simulink model "Ieee14_CC_2019b"  (R2019b)
settings: Solver=ode1  StartTime=0.0  StopTime=3600  FixedStep=1e-3  MaxStep=1e-4  RelTol=1e-3
model workspace (MAT data in the model file):
  pruebaValor = 0
libraries: powerlib x118, dspnetwork x116, source_mod x14, simulink x1
(part 1 of 3)
settings Model: NumberOfSteps=10  OrderedModelArguments=off  Creator=Mónica Alonso  LastModifiedBy=COSEC
settings DataIOCC: ReturnWorkspaceOutputs=off
settings OptimizationCC: LocalBlockOutputs=off
settings DebuggingCC: UnconnectedInputMsg=none  UnconnectedOutputMsg=none  UnconnectedLineMsg=none  ArithmeticOperatorsInVariantConditions=warning
settings SFSimCC: SimUseLocalCustomCode=off  CustomCodeUndefinedFunction=UseInterfaceOnly
settings RTWCC: RTWUseLocalCustomCode=off

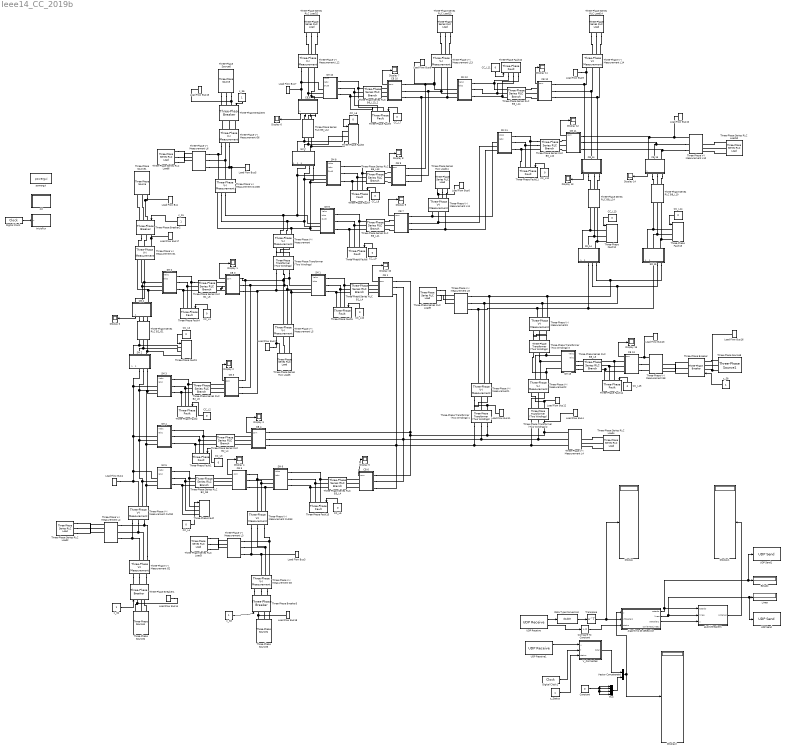
== system Ieee14_CC_2019b ==
  " ajustVBreakers" : MATLAB Function  TreatAsAtomicUnit=on
  "Algoritmo de deteccion " : MATLAB Function  TreatAsAtomicUnit=on
  CB 0 : Subsystem
  CB 1 : Subsystem
  CB 10 : Subsystem
  CB 11 : Subsystem
  CB 12 : Subsystem
  CB 13 : Subsystem
  CB 14 : Subsystem
  CB 15 : Subsystem
  CB 2 : Subsystem
  CB 3 : Subsystem
  CB 4 : Subsystem
  CB 5 : Subsystem
  CB 6 : Subsystem
  CB 7 : Subsystem
  CB 8 : Subsystem
  CB 9 : Subsystem
  CC : MATLAB Function  TreatAsAtomicUnit=on
  CC_L{0..15} (16 alike) : Constant  Value=0
  Compare To Constant : simulink/Logic and Bit Operations/Compare To Constant  relop=>  const=0  OutDataTypeStr=boolean
  Constant : Constant  Value=0
  Data Type Conversion : DataTypeConversion  OutDataTypeStr=double
  Digital Clock : DigitalClock  SampleTime=1e-1
  Digital Clock1 : DigitalClock  SampleTime=1e-3
  Display : Display
  Display {0..15} (16 alike) : Display
      settings: Format=decimal (Stored Integer)
  Display1 : Display
  Display2 : Display
  Estado : Display
  InicioFcn : MATLAB Function  TreatAsAtomicUnit=on
  Linea : Display
  Load Flow Bus : powerlib/Measurements/Load Flow Bus  LConnTagsString=a  Phases=single  Connectors=on one side  ID=BUS_G1  Vbase=69e3  Vref=1.06  Vangle=0  VLF=1.06  VLFb=1  VLFc=1  angleLF=0  angleLFb=0  angleLFc=0
      settings: SourceProductName=Simscape Electrical
  Load Flow Bus1 : powerlib/Measurements/Load Flow Bus  LConnTagsString=a  Phases=single  Connectors=on one side  ID=BUS_2  Vbase=69e3  Vref=1.045  Vangle=0  VLF=1.045  VLFb=1  VLFc=1  angleLF=-0.4295  angleLFb=0  angleLFc=0
      settings: SourceProductName=Simscape Electrical
  Load Flow Bus10 : powerlib/Measurements/Load Flow Bus  LConnTagsString=a  Phases=single  Connectors=on one side  ID=BUS_10  Vbase=13.8e3  Vref=1  Vangle=0  VLF=1.028  VLFb=1  VLFc=1  angleLF=-4.763  angleLFb=0  angleLFc=0
      settings: SourceProductName=Simscape Electrical
  Load Flow Bus11 : powerlib/Measurements/Load Flow Bus  LConnTagsString=a  Phases=single  Connectors=on one side  ID=BUS_9  Vbase=13.8e3  Vref=1  Vangle=0  VLF=1.042  VLFb=1  VLFc=1  angleLF=-4.02  angleLFb=0  angleLFc=0
      settings: SourceProductName=Simscape Electrical
  Load Flow Bus12 : powerlib/Measurements/Load Flow Bus  LConnTagsString=a  Phases=single  Connectors=on one side  ID=BUS_7  Vbase=18e3  Vref=1  Vangle=0  VLF=1.042  VLFb=1  VLFc=1  angleLF=-3.998  angleLFb=0  angleLFc=0
      settings: SourceProductName=Simscape Electrical
  Load Flow Bus13 : powerlib/Measurements/Load Flow Bus  LConnTagsString=a  Phases=single  Connectors=on one side  ID=BUS_8  Vbase=18e3  Vref=1.09  Vangle=0  VLF=1.082  VLFb=1  VLFc=1  angleLF=-4.037  angleLFb=0  angleLFc=0
      settings: SourceProductName=Simscape Electrical
  Load Flow Bus14 : powerlib/Measurements/Load Flow Bus  LConnTagsString=a  Phases=single  Connectors=on one side  ID=BUS_G2  Vbase=69e3  Vref=1.045  Vangle=0  VLF=1.045  VLFb=1  VLFc=1  angleLF=-0.435  angleLFb=0  angleLFc=0
      settings: SourceProductName=Simscape Electrical
  Load Flow Bus15 : powerlib/Measurements/Load Flow Bus  LConnTagsString=a  Phases=single  Connectors=on one side  ID=BUS_G6  Vbase=13.8e3  Vref=1.07  Vangle=0  VLF=1.07  VLFb=1  VLFc=1  angleLF=-4.448  angleLFb=0  angleLFc=0
      settings: SourceProductName=Simscape Electrical
  Load Flow Bus16 : powerlib/Measurements/Load Flow Bus  LConnTagsString=a  Phases=single  Connectors=on one side  ID=BUS_G8  Vbase=18e3  Vref=1.09  Vangle=0  VLF=1.082  VLFb=1  VLFc=1  angleLF=-4.074  angleLFb=0  angleLFc=0
      settings: SourceProductName=Simscape Electrical
  Load Flow Bus17 : powerlib/Measurements/Load Flow Bus  LConnTagsString=a  Phases=single  Connectors=on one side  ID=BUS_1  Vbase=69e3  Vref=1.06  Vangle=0  VLF=1.06  VLFb=1  VLFc=1  angleLF=0.000603  angleLFb=0  angleLFc=0
      settings: SourceProductName=Simscape Electrical
  Load Flow Bus18 : powerlib/Measurements/Load Flow Bus  LConnTagsString=a  Phases=single  Connectors=on one side  ID=BUS_G3  Vbase=69e3  Vref=1.01  Vangle=0  VLF=1.029  VLFb=1  VLFc=1  angleLF=-1.19  angleLFb=0  angleLFc=0
      settings: SourceProductName=Simscape Electrical
  Load Flow Bus2 : powerlib/Measurements/Load Flow Bus  LConnTagsString=a  Phases=single  Connectors=on one side  ID=BUS_5  Vbase=69e3  Vref=1  Vangle=0  VLF=1.008  VLFb=1  VLFc=1  angleLF=-3.193  angleLFb=0  angleLFc=0
      settings: SourceProductName=Simscape Electrical
  Load Flow Bus3 : powerlib/Measurements/Load Flow Bus  LConnTagsString=a  Phases=single  Connectors=on one side  ID=BUS_3  Vbase=69e3  Vref=1.01  Vangle=0  VLF=1.029  VLFb=1  VLFc=1  angleLF=-1.19  angleLFb=0  angleLFc=0
      settings: SourceProductName=Simscape Electrical
  Load Flow Bus4 : powerlib/Measurements/Load Flow Bus  LConnTagsString=a  Phases=single  Connectors=on one side  ID=BUS_4  Vbase=69e3  Vref=1  Vangle=0  VLF=1.013  VLFb=1  VLFc=1  angleLF=-3.392  angleLFb=0  angleLFc=0
      settings: SourceProductName=Simscape Electrical
  Load Flow Bus5 : powerlib/Measurements/Load Flow Bus  LConnTagsString=a  Phases=single  Connectors=on one side  ID=BUS_6  Vbase=13.8e3  Vref=1.07  Vangle=0  VLF=1.07  VLFb=1  VLFc=1  angleLF=-4.411  angleLFb=0  angleLFc=0
      settings: SourceProductName=Simscape Electrical
  Load Flow Bus6 : powerlib/Measurements/Load Flow Bus  LConnTagsString=a  Phases=single  Connectors=on one side  ID=BUS_11  Vbase=13.8e3  Vref=1  Vangle=0  VLF=1.029  VLFb=1  VLFc=1  angleLF=-5.425  angleLFb=0  angleLFc=0
      settings: SourceProductName=Simscape Electrical
  Load Flow Bus7 : powerlib/Measurements/Load Flow Bus  LConnTagsString=a  Phases=single  Connectors=on one side  ID=BUS_12  Vbase=13.8e3  Vref=1  Vangle=0  VLF=1.034  VLFb=1  VLFc=1  angleLF=-5.514  angleLFb=0  angleLFc=0
      settings: SourceProductName=Simscape Electrical
  Load Flow Bus8 : powerlib/Measurements/Load Flow Bus  LConnTagsString=a  Phases=single  Connectors=on one side  ID=BUS_13  Vbase=13.8e3  Vref=1  Vangle=0  VLF=1.036  VLFb=1  VLFc=1  angleLF=-5.353  angleLFb=0  angleLFc=0
      settings: SourceProductName=Simscape Electrical
  Load Flow Bus9 : powerlib/Measurements/Load Flow Bus  LConnTagsString=a  Phases=single  Connectors=on one side  ID=BUS_14  Vbase=13.8e3  Vref=1  Vangle=0  VLF=1.013  VLFb=1  VLFc=1  angleLF=-5.548  angleLFb=0  angleLFc=0
      settings: SourceProductName=Simscape Electrical
  Mux : Mux
  SM 0 : Subsystem
  SM 1 : Subsystem
  SM 10 : Subsystem
  SM 11 : Subsystem
  SM 12 : Subsystem
  SM 13 : Subsystem
  SM 14 : Subsystem
  SM 15 : Subsystem
  SM 2 : Subsystem
  SM 3 : Subsystem
  SM 4 : Subsystem
  SM 5 : Subsystem
  SM 6 : Subsystem
  SM 7 : Subsystem
  SM 8 : Subsystem
  SM 9 : Subsystem
  Three-Phase Series RLC B1_L4 : powerlib/Elements/Three-Phase Series RLC Branch  LConnTagsString=A|B|C  RConnTagsString=A|B|C  BranchType=RL  Resistance=0.01335*47.61  Inductance=0.04211*47.61/(100*pi)  Capacitance=100*pi/0.034  Measurements=None
      settings: SourceProductName=Simscape Electrical
  Three-Phase Series RLC B1_L5 : powerlib/Elements/Three-Phase Series RLC Branch  LConnTagsString=A|B|C  RConnTagsString=A|B|C  BranchType=RLC  Resistance=0.05403*47.61  Inductance=0.22304*47.61/(100*pi)  Capacitance=1/(0.0492*47.61*100*pi)  Measurements=None
      settings: SourceProductName=Simscape Electrical
  Three-Phase Series RLC B2_G1 : powerlib/Elements/Three-Phase Series RLC Branch  LConnTagsString=A|B|C  RConnTagsString=A|B|C  BranchType=RLC  Resistance=0.01938*47.61  Inductance=0.05917*47.61/(100*pi)  Capacitance=1/(0.0528*47.61*100*pi)  Measurements=None
      settings: SourceProductName=Simscape Electrical
  Three-Phase Series RLC B2_G3 : powerlib/Elements/Three-Phase Series RLC Branch  LConnTagsString=A|B|C  RConnTagsString=A|B|C  BranchType=RLC  Resistance=0.04699*47.61  Inductance=0.19797*47.61/(100*pi)  Capacitance=1/(0.0438*47.61*100*pi)  Measurements=None
      settings: SourceProductName=Simscape Electrical
  Three-Phase Series RLC B2_L4 : powerlib/Elements/Three-Phase Series RLC Branch  LConnTagsString=A|B|C  RConnTagsString=A|B|C  BranchType=RLC  Resistance=0.05811*47.61  Inductance=0.17632*47.61/(100*pi)  Capacitance=1/(0.034*47.61*100*pi)  Measurements=None
      settings: SourceProductName=Simscape Electrical
  Three-Phase Series RLC B2_L5 : powerlib/Elements/Three-Phase Series RLC Branch  LConnTagsString=A|B|C  RConnTagsString=A|B|C  BranchType=RLC  Resistance=0.05695*47.61  Inductance=0.17388*47.61/(100*pi)  Capacitance=1/(0.0346*47.61*100*pi)  Measurements=None
      settings: SourceProductName=Simscape Electrical
  Three-Phase Series RLC B3_L4 : powerlib/Elements/Three-Phase Series RLC Branch  LConnTagsString=A|B|C  RConnTagsString=A|B|C  BranchType=RLC  Resistance=0.06701*47.61  Inductance=0.17103*47.61/(100*pi)  Capacitance=1/(0.0128*47.61*100*pi)  Measurements=None
      settings: SourceProductName=Simscape Electrical
  Three-Phase Series RLC B6_L10 : powerlib/Elements/Three-Phase Series RLC Branch  LConnTagsString=A|B|C  RConnTagsString=A|B|C  BranchType=RL  Resistance=0.17093*1.9044  Inductance=0.34802*1.9044/(100*pi)  Capacitance=100*pi/0.034  Measurements=None
      settings: SourceProductName=Simscape Electrical
  Three-Phase Series RLC B6_L11 : powerlib/Elements/Three-Phase Series RLC Branch  LConnTagsString=A|B|C  RConnTagsString=A|B|C  BranchType=RL  Resistance=0.09498*1.9044  Inductance=0.1989*1.9044/(100*pi)  Capacitance=100*pi/0.034  Measurements=None
      settings: SourceProductName=Simscape Electrical
  Three-Phase Series RLC B6_L12 : powerlib/Elements/Three-Phase Series RLC Branch  LConnTagsString=A|B|C  RConnTagsString=A|B|C  BranchType=RL  Resistance=0.12291*1.9044  Inductance=0.25581*1.9044/(100*pi)  Capacitance=100*pi/0.034  Measurements=None
      settings: SourceProductName=Simscape Electrical
  Three-Phase Series RLC B6_L13 : powerlib/Elements/Three-Phase Series RLC Branch  LConnTagsString=A|B|C  RConnTagsString=A|B|C  BranchType=RL  Resistance=0.06615*1.9044  Inductance=0.13027*1.9044/(100*pi)  Capacitance=100*pi/0.034  Measurements=None
      settings: SourceProductName=Simscape Electrical
  Three-Phase Series RLC B6_L13_2 : powerlib/Elements/Three-Phase Series RLC Branch  LConnTagsString=A|B|C  RConnTagsString=A|B|C  BranchType=RL  Resistance=0.06615*1.9044  Inductance=0.13027*1.9044/(100*pi)  Capacitance=100*pi/0.034  Measurements=None
      settings: SourceProductName=Simscape Electrical
  Three-Phase Series RLC B6_L14 : powerlib/Elements/Three-Phase Series RLC Branch  LConnTagsString=A|B|C  RConnTagsString=A|B|C  BranchType=RL  Resistance=0.17093*1.9044  Inductance=0.34802*1.9044/(100*pi)  Capacitance=100*pi/0.034  Measurements=None
      settings: SourceProductName=Simscape Electrical
  Three-Phase Series RLC B8_L10 : powerlib/Elements/Three-Phase Series RLC Branch  LConnTagsString=A|B|C  RConnTagsString=A|B|C  BranchType=RL  Resistance=0.03181*1.9044  Inductance=0.0845*1.9044/(100*pi)  Capacitance=100*pi/0.034  Measurements=None
      settings: SourceProductName=Simscape Electrical
  Three-Phase Series RLC B8_L14 : powerlib/Elements/Three-Phase Series RLC Branch  LConnTagsString=A|B|C  RConnTagsString=A|B|C  BranchType=RL  Resistance=0.12711*1.9044  Inductance=0.27038*1.9044/(100*pi)  Capacitance=100*pi/0.034  Measurements=None
      settings: SourceProductName=Simscape Electrical
  Three-Phase Series RLC B8_L5 : powerlib/Elements/Three-Phase Series RLC Branch  LConnTagsString=A|B|C  RConnTagsString=A|B|C  BranchType=L  Resistance=0  Inductance=0.17615*3.24/(100*pi)  Capacitance=100*pi/0.034  Measurements=None
      settings: SourceProductName=Simscape Electrical
  Three-Phase Series RLC Load10 : source_mod/Three-Phase Series RLC Load  LConnTagsString=A|B|C  Configuration=Y (grounded)  NominalVoltage=(13800)*1.028  Vabc=[1e3 1e3 1e3]  Vabcp=[1e3 1e3 1e3]  NominalFrequency=50  UnbalancedPower=off  ActivePower=17472840  InductivePower=10226040  CapacitivePower=100  Pabc=[10e3 9e3 11e3]  QLabc=[100 90 110]  QCabc=[100 90 110]  Pabcp=[10e3 9e3 11e3]  QLabcp=[100 90 110]  QCabcp=[100 90 110]  Measurements=Branch voltages and currents  LoadType=constant PQ
      settings: AttributesFormatString=\n  SourceProductName=my library
  Three-Phase Series RLC Load11 : source_mod/Three-Phase Series RLC Load  LConnTagsString=A|B|C  Configuration=Y (grounded)  NominalVoltage=(13800)*1.02933  Vabc=[1e3 1e3 1e3]  Vabcp=[1e3 1e3 1e3]  NominalFrequency=50  UnbalancedPower=off  ActivePower=14912240  InductivePower=8727440  CapacitivePower=0  Pabc=[10e3 9e3 11e3]  QLabc=[100 90 110]  QCabc=[100 90 110]  Pabcp=[10e3 9e3 11e3]  QLabcp=[100 90 110]  QCabcp=[100 90 110]  Measurements=Branch voltages and currents  LoadType=constant PQ
      settings: AttributesFormatString=\n  SourceProductName=my library
  Three-Phase Series RLC Load12 : source_mod/Three-Phase Series RLC Load  LConnTagsString=A|B|C  Configuration=Y (grounded)  NominalVoltage=(13800)*1.03362  Vabc=[1e3 1e3 1e3]  Vabcp=[1e3 1e3 1e3]  NominalFrequency=50  UnbalancedPower=off  ActivePower=14706090  InductivePower=8606790  CapacitivePower=100  Pabc=[10e3 9e3 11e3]  QLabc=[100 90 110]  QCabc=[100 90 110]  Pabcp=[10e3 9e3 11e3]  QLabcp=[100 90 110]  QCabcp=[100 90 110]  Measurements=Branch voltages and currents  LoadType=constant PQ
      settings: AttributesFormatString=\n  SourceProductName=my library
  Three-Phase Series RLC Load13 : source_mod/Three-Phase Series RLC Load  LConnTagsString=A|B|C  Configuration=Y (grounded)  NominalVoltage=(13800)*1.03599  Vabc=[1e3 1e3 1e3]  Vabcp=[1e3 1e3 1e3]  NominalFrequency=50  UnbalancedPower=off  ActivePower=18199790  InductivePower=10651490  CapacitivePower=100  Pabc=[10e3 9e3 11e3]  QLabc=[100 90 110]  QCabc=[100 90 110]  Pabcp=[10e3 9e3 11e3]  QLabcp=[100 90 110]  QCabcp=[100 90 110]  Measurements=Branch voltages and currents  LoadType=constant PQ
      settings: AttributesFormatString=\n  SourceProductName=my library
  Three-Phase Series RLC Load14 : source_mod/Three-Phase Series RLC Load  LConnTagsString=A|B|C  Configuration=Y (grounded)  NominalVoltage=(13800)*1.01323  Vabc=[1e3 1e3 1e3]  Vabcp=[1e3 1e3 1e3]  NominalFrequency=50  UnbalancedPower=off  ActivePower=13888000  InductivePower=8128000  CapacitivePower=1  Pabc=[10e3 9e3 11e3]  QLabc=[100 90 110]  QCabc=[100 90 110]  Pabcp=[10e3 9e3 11e3]  QLabcp=[100 90 110]  QCabcp=[100 90 110]  Measurements=Branch voltages and currents  LoadType=constant PQ
      settings: AttributesFormatString=\n  SourceProductName=my library
  Three-Phase Series RLC Load2 : source_mod/Three-Phase Series RLC Load  LConnTagsString=A|B|C  Configuration=Y (grounded)  NominalVoltage=(69000)*1.04466  Vabc=[1e3 1e3 1e3]  Vabcp=[1e3 1e3 1e3]  NominalFrequency=50  UnbalancedPower=off  ActivePower=11817820  InductivePower=6916420  CapacitivePower=0  Pabc=15  QLabc=[100 90 110]  QCabc=[100 90 110]  Pabcp=[10e3 9e3 11e3]  QLabcp=[100 90 110]  QCabcp=[100 90 110]  Measurements=Branch voltages and currents  LoadType=constant PQ
      settings: AttributesFormatString=\n  SourceProductName=my library
  Three-Phase Series RLC Load3 : source_mod/Three-Phase Series RLC Load  LConnTagsString=A|B|C  Configuration=Y (grounded)  NominalVoltage=(69000)*1.02865  Vabc=[1e3 1e3 1e3]  Vabcp=[1e3 1e3 1e3]  NominalFrequency=50  UnbalancedPower=off  ActivePower=15090180  InductivePower=8831580  CapacitivePower=0  Pabc=[10e3 9e3 11e3]  QLabc=[100 90 110]  QCabc=[100 90 110]  Pabcp=[10e3 9e3 11e3]  QLabcp=[100 90 110]  QCabcp=[100 90 110]  Measurements=Branch voltages and currents  LoadType=constant PQ
      settings: AttributesFormatString=\n  SourceProductName=my library
  Three-Phase Series RLC Load4 : source_mod/Three-Phase Series RLC Load  LConnTagsString=A|B|C  Configuration=Y (grounded)  NominalVoltage=(69000)*1.0131  Vabc=[1e3 1e3 1e3]  Vabcp=[1e3 1e3 1e3]  NominalFrequency=50  UnbalancedPower=off  ActivePower=20484800  InductivePower=11988800  CapacitivePower=3.9e6  Pabc=[10e3 9e3 11e3]  QLabc=[100 90 110]  QCabc=[100 90 110]  Pabcp=[10e3 9e3 11e3]  QLabcp=[100 90 110]  QCabcp=[100 90 110]  Measurements=Branch voltages and currents  LoadType=constant PQ
      settings: AttributesFormatString=\n  SourceProductName=my library
  Three-Phase Series RLC Load5 : source_mod/Three-Phase Series RLC Load  LConnTagsString=A|B|C  Configuration=Y (grounded)  NominalVoltage=(69000)*1.00791  Vabc=[1e3 1e3 1e3]  Vabcp=[1e3 1e3 1e3]  NominalFrequency=50  UnbalancedPower=off  ActivePower=19805590  InductivePower=11591290  CapacitivePower=0  Pabc=[10e3 9e3 11e3]  QLabc=[100 90 110]  QCabc=[100 90 110]  Pabcp=[10e3 9e3 11e3]  QLabcp=[100 90 110]  QCabcp=[100 90 110]  Measurements=Branch voltages and currents  LoadType=constant PQ
      settings: AttributesFormatString=\n  SourceProductName=my library
  Three-Phase Series RLC Load6 : source_mod/Three-Phase Series RLC Load  LConnTagsString=A|B|C  Configuration=Y (grounded)  NominalVoltage=(13800)*1.07  Vabc=[1e3 1e3 1e3]  Vabcp=[1e3 1e3 1e3]  NominalFrequency=50  UnbalancedPower=off  ActivePower=16845710  InductivePower=9859010  CapacitivePower=0  Pabc=[10e3 9e3 11e3]  QLabc=[100 90 110]  QCabc=[100 90 110]  Pabcp=[10e3 9e3 11e3]  QLabcp=[100 90 110]  QCabcp=[100 90 110]  Measurements=Branch voltages and currents  LoadType=constant PQ
      settings: AttributesFormatString=\n  SourceProductName=my library
  Three-Phase Series RLC Load9 : source_mod/Three-Phase Series RLC Load  LConnTagsString=A|B|C  Configuration=Y (grounded)  NominalVoltage=(13800)*1.04242  Vabc=[1e3 1e3 1e3]  Vabcp=[1e3 1e3 1e3]  NominalFrequency=50  UnbalancedPower=off  ActivePower=12028310  InductivePower=7039610  CapacitivePower=19e6  Pabc=[10e3 9e3 11e3]  QLabc=[100 90 110]  QCabc=[100 90 110]  Pabcp=[10e3 9e3 11e3]  QLabcp=[100 90 110]  QCabcp=[100 90 110]  Measurements=Branch voltages and currents  LoadType=constant PQ
      settings: AttributesFormatString=\n  SourceProductName=my library
  Three-Phase Transformer (Two Windings) : powerlib/Elements/Three-Phase Transformer (Two Windings)  Winding1Connection=Yg  Winding2Connection=Yg  CoreType=Three single-phase transformers  SetSaturation=off  Hysteresis=off  DataFile='hysteresis'  SetInitialFlux=off  Measurements=None  UNITS=pu  NominalPower=[ 100e6 , 50 ]  Winding1="[13.8e3 , 0 ,  0]"  Winding2=[69e3*0.932, 0 ,0.25202*47.61/(100*pi) ]  Rm=500  Lm=500  L0=0.5  Saturation=[ 0,0 ; 0.0024,1.2 ; 1.0,1.52 ]  InitialFluxes=[ 0.8 , -0.8 , 0.7 ]  BreakLoop=off  DiscreteSolver=Trapezoidal iterative  DataType=off  TransfoNumber=1
      settings: SourceProductName=Simscape Electrical
  Three-Phase Transformer (Two Windings)1 : powerlib/Elements/Three-Phase Transformer (Two Windings)  Winding1Connection=Yg  Winding2Connection=Yg  CoreType=Three single-phase transformers  SetSaturation=off  Hysteresis=off  DataFile='hysteresis'  SetInitialFlux=off  Measurements=None  UNITS=pu  NominalPower=[ 100e6 , 50 ]  Winding1=[13.8e3 , 0 , 0 ]  Winding2=[69e3*0.969, 0 , 0.55618*47.61/(100*pi)]  Rm=500  Lm=500  L0=0.5  Saturation=[ 0,0 ; 0.0024,1.2 ; 1.0,1.52 ]  InitialFluxes=[ 0.8 , -0.8 , 0.7 ]  BreakLoop=off  DiscreteSolver=Trapezoidal iterative  DataType=off  TransfoNumber=1
      settings: SourceProductName=Simscape Electrical
  Three-Phase Transformer (Two Windings)2 : powerlib/Elements/Three-Phase Transformer (Two Windings)  Winding1Connection=Yg  Winding2Connection=Yg  CoreType=Three single-phase transformers  SetSaturation=off  Hysteresis=off  DataFile='hysteresis'  SetInitialFlux=off  Measurements=None  UNITS=pu  NominalPower=[ 100e6 , 50 ]  Winding1=[18e3 , 0 , 0]  Winding2=[69e3*0.978 , 0 ,0.20912*47.61/(100*pi)]  Rm=500  Lm=500  L0=0.5  Saturation=[ 0,0 ; 0.0024,1.2 ; 1.0,1.52 ]  InitialFluxes=[ 0.8 , -0.8 , 0.7 ]  BreakLoop=off  DiscreteSolver=Trapezoidal iterative  DataType=off  TransfoNumber=1
      settings: SourceProductName=Simscape Electrical
  Three-Phase Transformer (Two Windings)3 : powerlib/Elements/Three-Phase Transformer (Two Windings)  Winding1Connection=Yg  Winding2Connection=Yg  CoreType=Three single-phase transformers  SetSaturation=off  Hysteresis=off  DataFile='hysteresis'  SetInitialFlux=off  Measurements=None  UNITS=pu  NominalPower=[ 100e6 , 50 ]  Winding1=[13.8e3 , 0 , 0]  Winding2=[18e3, 0 ,0.11*3.24/(100*pi)]  Rm=500  Lm=500  L0=0.5  Saturation=[ 0,0 ; 0.0024,1.2 ; 1.0,1.52 ]  InitialFluxes=[ 0.8 , -0.8 , 0.7 ]  BreakLoop=off  DiscreteSolver=Trapezoidal iterative  DataType=off  TransfoNumber=1
      settings: SourceProductName=Simscape Electrical
  Three-Phase V-I Measurement{,1..3} (4 alike) : powerlib/Measurements/Three-Phase V-I Measurement  VoltageMeasurement=no  SetLabelV=off  LabelV=Vabc  Vpu=off  VpuLL=off  CurrentMeasurement=yes  SetLabelI=off  LabelI=Iabc  Ipu=off  Pbase=100e6  Vbase=500e3  OutputType=Complex  PhasorSimulation=off  PSBequivalent=0
      settings: SourceProductName=Simscape Electrical
  Three-Phase V-I Measurement G1 : powerlib/Measurements/Three-Phase V-I Measurement  VoltageMeasurement=phase-to-phase  SetLabelV=off  LabelV=Vabc  Vpu=off  VpuLL=off  CurrentMeasurement=yes  SetLabelI=off  LabelI=Iabc  Ipu=off  Pbase=100e6  Vbase=69e3  OutputType=Complex  PhasorSimulation=off  PSBequivalent=0
      settings: SourceProductName=Simscape Electrical
  Three-Phase V-I Measurement G2 : powerlib/Measurements/Three-Phase V-I Measurement  VoltageMeasurement=phase-to-ground  SetLabelV=off  LabelV=Vabc  Vpu=off  VpuLL=off  CurrentMeasurement=yes  SetLabelI=off  LabelI=Iabc  Ipu=off  Pbase=100e6  Vbase=69e3  OutputType=Complex  PhasorSimulation=off  PSBequivalent=0
      settings: SourceProductName=Simscape Electrical
  Three-Phase V-I Measurement G3 : powerlib/Measurements/Three-Phase V-I Measurement  VoltageMeasurement=phase-to-phase  SetLabelV=off  LabelV=Vabc  Vpu=off  VpuLL=off  CurrentMeasurement=yes  SetLabelI=off  LabelI=Iabc  Ipu=off  Pbase=100e6  Vbase=69e3  OutputType=Complex  PhasorSimulation=off  PSBequivalent=0
      settings: SourceProductName=Simscape Electrical
  Three-Phase V-I Measurement G6 : powerlib/Measurements/Three-Phase V-I Measurement  VoltageMeasurement=phase-to-phase  SetLabelV=off  LabelV=Vabc  Vpu=off  VpuLL=off  CurrentMeasurement=yes  SetLabelI=off  LabelI=Iabc  Ipu=off  Pbase=100e6  Vbase=13.8e3  OutputType=Complex  PhasorSimulation=off  PSBequivalent=0
      settings: SourceProductName=Simscape Electrical
  Three-Phase V-I Measurement G8 : powerlib/Measurements/Three-Phase V-I Measurement  VoltageMeasurement=phase-to-phase  SetLabelV=off  LabelV=Vabc  Vpu=off  VpuLL=off  CurrentMeasurement=yes  SetLabelI=off  LabelI=Iabc  Ipu=off  Pbase=100e6  Vbase=18e3  OutputType=Complex  PhasorSimulation=off  PSBequivalent=0
      settings: SourceProductName=Simscape Electrical
  Three-Phase V-I Measurement L{6,10..14} (6 alike) : powerlib/Measurements/Three-Phase V-I Measurement  VoltageMeasurement=phase-to-phase  SetLabelV=off  LabelV=Vabc  Vpu=off  VpuLL=off  CurrentMeasurement=yes  SetLabelI=off  LabelI=Iabc  Ipu=off  Pbase=100e6  Vbase=13.8e3  OutputType=Complex  PhasorSimulation=off  PSBequivalent=0
      settings: SourceProductName=Simscape Electrical
  Three-Phase V-I Measurement L2 : powerlib/Measurements/Three-Phase V-I Measurement  VoltageMeasurement=phase-to-ground  SetLabelV=off  LabelV=Vabc  Vpu=off  VpuLL=off  CurrentMeasurement=yes  SetLabelI=off  LabelI=Iabc  Ipu=off  Pbase=100e6  Vbase=69e3  OutputType=Complex  PhasorSimulation=off  PSBequivalent=0
      settings: SourceProductName=Simscape Electrical
  Three-Phase V-I Measurement L{3..5,9} (4 alike) : powerlib/Measurements/Three-Phase V-I Measurement  VoltageMeasurement=phase-to-phase  SetLabelV=off  LabelV=Vabc  Vpu=off  VpuLL=off  CurrentMeasurement=yes  SetLabelI=off  LabelI=Iabc  Ipu=off  Pbase=100e6  Vbase=69e3  OutputType=Complex  PhasorSimulation=off  PSBequivalent=0
      settings: SourceProductName=Simscape Electrical
  Three-Phase V-I Measurement OutG2 : powerlib/Measurements/Three-Phase V-I Measurement  VoltageMeasurement=phase-to-phase  SetLabelV=off  LabelV=Vabc  Vpu=on  VpuLL=off  CurrentMeasurement=yes  SetLabelI=off  LabelI=Iabc  Ipu=off  Pbase=100e6  Vbase=69e3  OutputType=Complex  PhasorSimulation=off  PSBequivalent=0
      settings: SourceProductName=Simscape Electrical
  Three-Phase V-I Measurement OutG3 : powerlib/Measurements/Three-Phase V-I Measurement  VoltageMeasurement=phase-to-phase  SetLabelV=off  LabelV=Vabc  Vpu=on  VpuLL=off  CurrentMeasurement=yes  SetLabelI=off  LabelI=Iabc  Ipu=off  Pbase=100e6  Vbase=69e3  OutputType=Complex  PhasorSimulation=off  PSBequivalent=0
      settings: SourceProductName=Simscape Electrical
  Three-Phase V-I Measurement OutG6 : powerlib/Measurements/Three-Phase V-I Measurement  VoltageMeasurement=phase-to-phase  SetLabelV=off  LabelV=Vabc  Vpu=on  VpuLL=off  CurrentMeasurement=yes  SetLabelI=off  LabelI=Iabc  Ipu=off  Pbase=100e6  Vbase=13.8e3  OutputType=Complex  PhasorSimulation=off  PSBequivalent=0
      settings: SourceProductName=Simscape Electrical
  Three-Phase Breaker : powerlib/Elements/Three-Phase Breaker  InitialState=closed  SwitchA=on  SwitchB=on  SwitchC=on  SwitchTimes=[1.5]  External=on  BreakerResistance=0.01  SnubberResistance=1e6  SnubberCapacitance=inf  Measurements=Breaker voltages and currents
      settings: SourceProductName=Simscape Electrical
  Three-Phase Breaker{1..3,6} (4 alike) : powerlib/Elements/Three-Phase Breaker  InitialState=closed  SwitchA=on  SwitchB=on  SwitchC=on  SwitchTimes=[1]  External=on  BreakerResistance=0.01  SnubberResistance=1e6  SnubberCapacitance=inf  Measurements=Breaker voltages and currents
      settings: SourceProductName=Simscape Electrical
  Three-Phase Fault{,1..15} (16 alike) : powerlib/Elements/Three-Phase Fault  InitialStates=0  FaultA=on  FaultB=on  FaultC=on  GroundFault=on  SwitchTimes="[1/60  5/60]"  External=on  SwitchStatus=NaN  FaultResistance=0.001  GroundResistance=0.01  SnubberResistance=1e6  SnubberCapacitance=inf  Measurements=Fault voltages and currents
      settings: SourceProductName=Simscape Electrical
  Three-Phase Source1 : powerlib/Electrical Sources/Three-Phase Source  InternalConnection=Yg  VoltagePhases=off  Voltage=(69000)*1.06  PhaseAngle=0  Voltage_phases=[25e3 25e3 25e3]/sqrt(3)  PhaseAngles_phases=[0 -120 +120]  Frequency=50  NonIdealSource=off  SpecifyImpedance=off  Resistance=0.8929  Inductance=16.58e-3  ShortCircuitLevel=100e6  BaseVoltage=69e3  XRratio=7  BusType=swing  Pref=10e3  Qref=0  Prefabc=[10e3, 10e3, 10e3]  Qrefabc=[0, 0, 0]  Qmin=-inf  Qmax=inf
      settings: SourceProductName=Simscape Electrical
  Three-Phase Source2 : source_mod/Three-Phase Source1  InternalConnection=Yg  VoltagePhases=off  Voltage=(69000)*1.04471  PhaseAngle=-0.43499  Voltage_phases=[25e3 25e3 25e3]/sqrt(3)  PhaseAngles_phases=[0 -120 +120]  Frequency=50  NonIdealSource=off  SpecifyImpedance=on  Resistance=0.8929  Inductance=16.58e-3  ShortCircuitLevel=100e6  BaseVoltage=69e3  XRratio=7  BusType=PV  Pref=27824000  Qref=0  Prefabc=[10e3, 10e3, 10e3]  Qrefabc=[0, 0, 0]  Qmin=-40e6  Qmax=50e6
      settings: SourceProductName=my library
  Three-Phase Source3 : source_mod/Three-Phase Source1  InternalConnection=Yg  VoltagePhases=off  Voltage=(69000)*1.02871  PhaseAngle=-1.19  Voltage_phases=[25e3 25e3 25e3]/sqrt(3)  PhaseAngles_phases=[0 -120 +120]  Frequency=50  NonIdealSource=off  SpecifyImpedance=on  Resistance=0.8929  Inductance=16.58e-3  ShortCircuitLevel=100e6  BaseVoltage=69e3  XRratio=7  BusType=PV  Pref=25076000  Qref=0  Prefabc=[10e3, 10e3, 10e3]  Qrefabc=[0, 0, 0]  Qmin=0  Qmax=40e6
      settings: SourceProductName=my library
  Three-Phase Source6 : powerlib/Electrical Sources/Three-Phase Source  InternalConnection=Yg  VoltagePhases=off  Voltage=(13800)*1.07  PhaseAngle=-4.4484  Voltage_phases=[25e3 25e3 25e3]/sqrt(3)  PhaseAngles_phases=[0 -120 +120]  Frequency=50  NonIdealSource=off  SpecifyImpedance=off  Resistance=0.8929  Inductance=16.58e-3  ShortCircuitLevel=100e6  BaseVoltage=13.8e3  XRratio=7  BusType=PV  Pref=0  Qref=0  Prefabc=[10e3, 10e3, 10e3]  Qrefabc=[0, 0, 0]  Qmin=-6e6  Qmax=24e6
      settings: SourceProductName=Simscape Electrical
  Three-Phase Source8 : source_mod/Three-Phase Source1  InternalConnection=Yg  VoltagePhases=off  Voltage=(18000)*1.08152  PhaseAngle=-4.0736  Voltage_phases=[25e3 25e3 25e3]/sqrt(3)  PhaseAngles_phases=[0 -120 +120]  Frequency=50  NonIdealSource=off  SpecifyImpedance=on  Resistance=0.8929  Inductance=16.58e-3  ShortCircuitLevel=100e6  BaseVoltage=69e3  XRratio=7  BusType=PV  Pref=0  Qref=0  Prefabc=[10e3, 10e3, 10e3]  Qrefabc=[0, 0, 0]  Qmin=-6e6  Qmax=24e6
      settings: SourceProductName=my library
  Transpose : Math  Operator=transpose  SignedPower=off  SaturateOnIntegerOverflow=on
  UDP Receive : dspnetwork/UDP Receive  localURL='0.0.0.0'  localPort=40000  remoteURL='0.0.0.0'  remotePort=-1  recvBufferSize=32  dims=16  signalDatatype=int16  isComplex=off  isVarSize=off  showBlockingTime=off  blockingTime=0  sampletime=1  blockPlatform=[]
      settings: SourceProductName=Simulink
  UDP Receive1 : dspnetwork/UDP Receive  localURL='0.0.0.0'  localPort=40001  remoteURL='0.0.0.0'  remotePort=-1  recvBufferSize=32  dims=16  signalDatatype=int16  isComplex=off  isVarSize=off  showBlockingTime=off  blockingTime=0  sampletime=1  blockPlatform=[]
      settings: SourceProductName=Simulink
  UDP Send : dspnetwork/UDP Send  remoteURL='10.0.255.255'  remotePort=40002  localURL='0.0.0.0'  localPortSource=Automatically determine  localPort=-1  sampletime=-1  blockPlatform=[]  separateLengthPort=0
      settings: SourceProductName=Simulink
  UDP Send1 : dspnetwork/UDP Send  remoteURL='10.0.255.255'  remotePort=40003  localURL='0.0.0.0'  localPortSource=Automatically determine  localPort=-1  sampletime=-1  blockPlatform=[]  separateLengthPort=0
      settings: SourceProductName=Simulink
  V_Corrientes : MATLAB Function  TreatAsAtomicUnit=on
  Vector Concatenate : Concatenate
  c_S{1..3,6,8} (5 alike) : Constant
  c_Status : Constant
  powergui : powerlib/powergui  Priority=1  SimulationMode=Discrete  SampleTime=1e-3  frequency=50  Iterations=50  frequencyindice=0  Pbase=100e6  ErrMax=0.0001  UnitsV=kV  UnitsW=MW  buscounter=0  FunctionMessages=off  echomessages=off  EnableUseOfTLC=off  CurrentSourceSwitches=off  DisableSnubberDevices=off  DisableRonSwitches=off  DisableVfSwitches=off  DisplayEquations=off  AutomaticDiscreteSolvers=off  SolverType=Tustin/Backward Euler (TBE)  Interpol=off  ExternalGateDelay=off  methode=off  Ts=100  x0status=steady  SPID=on  SwTol=0  HookPort=off  NonlinearTolerance=1e-4  nMaxIteration=100  ContinueOnMaxIteration=off  RestoreLinks=warning  ResistiveCurrentMeasurement=off  Frange=[0:2:500]  Ylog=off  Xlog=on  ShowGrid=off  save=off  variable=ZData  structure=0  ZoomFFT=off  StartTime=0.0  cycles=1  DisplayStyle=1  fundamental=60  FreqAxis=off  MaxFrequency=1000  frequencyindicesteady=1  RmsSteady=1  display=off
      settings: SourceProductName=Simscape Electrical
  wires:
  CB 8/1(com) -> Display 6/1
  CB 11/1(com) -> Display 12/1
  CB 7/1(com) -> Display 9/1
  CB 1/1(com) -> Display 10/1
  CB 9/1(com) -> Display 8/1
  CB 5/1(com) -> Display 4/1
  CB 10/1(com) -> Display 7/1
  CB 2/1(com) -> Display 0/1
  CB 12/1(com) -> Display 11/1
  CB 3/1(com) -> Display 2/1
  CB 6/1(com) -> Display 5/1
  CB 4/1(com) -> Display 3/1
  CB 14/1(com) -> Display 13/1
  CB 15/1(com) -> Display 14/1
  CB 13/1(com) -> Display 15/1
  CB 0/1(com) -> Display 1/1
  Digital Clock/1 -> InicioFcn/1(u)
  CC_L5/1 -> Three-Phase Fault15/1
  CC_L15/1 -> Three-Phase Fault14/1
  CC_L14/1 -> Three-Phase Fault13/1
  CC_L13/1 -> Three-Phase Fault12/1
  CC_L12/1 -> Three-Phase Fault11/1
  CC_L11/1 -> Three-Phase Fault10/1
  CC_L7/1 -> Three-Phase Fault9/1
  CC_L6/1 -> Three-Phase Fault8/1
  CC_L8/1 -> Three-Phase Fault7/1
  CC_L9/1 -> Three-Phase Fault6/1
  CC_L10/1 -> Three-Phase Fault5/1
  CC_L1/1 -> Three-Phase Fault4/1
  CC_L0/1 -> Three-Phase Fault3/1
  CC_L2/1 -> Three-Phase Fault2/1
  CC_L3/1 -> Three-Phase Fault1/1
  CC_L4/1 -> Three-Phase Fault/1
  c_S8/1 -> Three-Phase Breaker/1
  c_S1/1 -> Three-Phase Breaker2/1
  c_S2/1 -> Three-Phase Breaker1/1
  c_S6/1 -> Three-Phase Breaker6/1
  c_S3/1 -> Three-Phase Breaker3/1
  " ajustVBreakers"/1(ordenes) -> Display1/1
  UDP Receive/2 -> Compare To Constant/1
  UDP Receive1/1 -> V_Corrientes/1(u)
  UDP Receive/1 -> Data Type Conversion/1
  "Algoritmo de deteccion "/3(vBreakers) -> " ajustVBreakers"/3(u)
  "Algoritmo de deteccion "/1(estado) -> UDP Send1/1, Estado/1, " ajustVBreakers"/1(estado)
  "Algoritmo de deteccion "/2(linea) -> UDP Send/1, Linea/1, " ajustVBreakers"/2(linea)
  c_Status/1 -> V_Corrientes/3(status)
  Digital Clock1/1 -> V_Corrientes/2(t)
  Compare To Constant/1 -> "Algoritmo de deteccion "/3(status)
  Data Type Conversion/1 -> Transpose/1
  Transpose/1 -> Display/1, "Algoritmo de deteccion "/2("vBreakers ")
  V_Corrientes/1(total) -> Vector Concatenate/1
  Vector Concatenate/1 -> "Algoritmo de deteccion "/1(u), Display2/1
  Constant/1 -> Mux/1, Mux/2, Mux/3, Mux/4
  Mux/1 -> Vector Concatenate/2
  connections:
  Three-Phase Transformer (Two Windings)3/LConn3 -- Three-Phase V-I Measurement3/LConn3
  Three-Phase Transformer (Two Windings)3/LConn2 -- Three-Phase V-I Measurement3/LConn2
  Three-Phase V-I Measurement3/LConn1 -- Three-Phase Transformer (Two Windings)3/LConn1
  Three-Phase Transformer (Two Windings)2/LConn3 -- Three-Phase V-I Measurement2/LConn3
  Three-Phase Transformer (Two Windings)2/LConn2 -- Three-Phase V-I Measurement2/LConn2
  SM 13/LConn1 -- Three-Phase V-I Measurement2/RConn1 -- Three-Phase Transformer (Two Windings)3/RConn1
  Three-Phase Transformer (Two Windings)1/LConn3 -- Three-Phase V-I Measurement1/LConn3
  Three-Phase Transformer (Two Windings)1/LConn2 -- Three-Phase V-I Measurement1/LConn2
  Load Flow Bus11/LConn1 -- Three-Phase V-I Measurement1/LConn1 -- Three-Phase Transformer (Two Windings)1/LConn1
  Three-Phase Transformer (Two Windings)/LConn3 -- Three-Phase V-I Measurement/LConn3
  Three-Phase Transformer (Two Windings)/LConn2 -- Three-Phase V-I Measurement/LConn2
  Three-Phase V-I Measurement/LConn1 -- Three-Phase Transformer (Two Windings)/LConn1
  Three-Phase Breaker2/RConn1 -- Three-Phase V-I Measurement G1/LConn1 -- Load Flow Bus17/LConn1
  Three-Phase Breaker2/LConn1 -- Three-Phase Source1/RConn1 -- Load Flow Bus/LConn1
  Three-Phase Breaker2/LConn2 -- Three-Phase Source1/RConn2
  Three-Phase V-I Measurement G1/LConn2 -- Three-Phase Breaker2/RConn2
  Three-Phase Breaker2/RConn3 -- Three-Phase V-I Measurement G1/LConn3
  Three-Phase Breaker2/LConn3 -- Three-Phase Source1/RConn3
  Three-Phase V-I Measurement L10/LConn3 -- CB 15/LConn3 -- CB 11/LConn3
  Three-Phase V-I Measurement L10/LConn2 -- CB 15/LConn2 -- CB 11/LConn2
  CB 11/RConn3 -- Three-Phase Series RLC B6_L10/RConn3
  CB 11/RConn2 -- Three-Phase Series RLC B6_L10/RConn2
  CB 11/RConn1 -- Three-Phase Series RLC B6_L10/RConn1
  CB 12/LConn3 -- Three-Phase V-I Measurement L14/LConn3 -- CB 14/LConn3
  CB 12/LConn2 -- Three-Phase V-I Measurement L14/LConn2 -- CB 14/LConn2
  CB 12/RConn3 -- Three-Phase Series RLC B6_L14/RConn3
  CB 12/RConn2 -- Three-Phase Series RLC B6_L14/RConn2
  CB 12/RConn1 -- Three-Phase Series RLC B6_L14/RConn1
  CB 10/RConn3 -- Three-Phase Series RLC B6_L13_2/RConn3
  CB 10/RConn2 -- Three-Phase Series RLC B6_L13_2/RConn2
  CB 10/RConn1 -- Three-Phase Series RLC B6_L13_2/RConn1
  CB 8/RConn3 -- Three-Phase Series RLC B6_L12/RConn3
  CB 8/RConn2 -- Three-Phase Series RLC B6_L12/RConn2
  CB 8/RConn1 -- Three-Phase Series RLC B6_L12/RConn1
  CB 9/RConn3 -- Three-Phase Series RLC B6_L13/LConn3
  CB 9/RConn2 -- Three-Phase Series RLC B6_L13/LConn2
  CB 9/RConn1 -- Three-Phase Series RLC B6_L13/LConn1
  CB 7/RConn3 -- Three-Phase Series RLC B6_L11/RConn3
  CB 7/RConn2 -- Three-Phase Series RLC B6_L11/RConn2
  CB 7/RConn1 -- Three-Phase Series RLC B6_L11/RConn1
  CB 15/RConn3 -- Three-Phase Series RLC B8_L10/RConn3
  CB 15/RConn2 -- Three-Phase Series RLC B8_L10/RConn2
  CB 15/RConn1 -- Three-Phase Series RLC B8_L10/RConn1
  CB 14/RConn3 -- Three-Phase Series RLC B8_L14/RConn3
  CB 14/RConn2 -- Three-Phase Series RLC B8_L14/RConn2
  CB 14/RConn1 -- Three-Phase Series RLC B8_L14/RConn1
  CB 13/LConn3 -- Three-Phase V-I Measurement G8/LConn3
  CB 13/LConn2 -- Three-Phase V-I Measurement G8/LConn2
  Three-Phase Fault14/LConn3 -- CB 13/RConn3 -- Three-Phase Series RLC B8_L5/RConn3
  Three-Phase Fault14/LConn2 -- CB 13/RConn2 -- Three-Phase Series RLC B8_L5/RConn2
  Three-Phase Fault14/LConn1 -- CB 13/RConn1 -- Three-Phase Series RLC B8_L5/RConn1
  CB 1/RConn3 -- Three-Phase Series RLC B1_L4/RConn3
  CB 1/RConn2 -- Three-Phase Series RLC B1_L4/RConn2
  CB 1/RConn1 -- Three-Phase Series RLC B1_L4/RConn1
  CB 2/RConn3 -- Three-Phase Series RLC B2_G1/RConn3
  CB 2/RConn2 -- Three-Phase Series RLC B2_G1/RConn2
  CB 2/RConn1 -- Three-Phase Series RLC B2_G1/RConn1
  CB 0/RConn2 -- Three-Phase Series RLC B1_L5/RConn3
  CB 0/RConn3 -- Three-Phase Series RLC B1_L5/RConn2
  CB 0/RConn1 -- Three-Phase Series RLC B1_L5/RConn1
  CB 3/RConn3 -- Three-Phase Series RLC B2_L5/RConn3
  CB 3/RConn2 -- Three-Phase Series RLC B2_L5/RConn2
  CB 3/RConn1 -- Three-Phase Series RLC B2_L5/RConn1
  CB 4/RConn3 -- Three-Phase Series RLC B2_L4/RConn3
  CB 4/RConn2 -- Three-Phase Series RLC B2_L4/RConn2
  CB 4/RConn1 -- Three-Phase Series RLC B2_L4/RConn1
  CB 6/RConn3 -- Three-Phase Series RLC B3_L4/RConn3
  CB 6/RConn2 -- Three-Phase Series RLC B3_L4/RConn2
  CB 6/RConn1 -- Three-Phase Series RLC B3_L4/RConn1
  CB 5/RConn3 -- Three-Phase Series RLC B2_G3/RConn3
  CB 5/RConn2 -- Three-Phase Series RLC B2_G3/RConn2
  CB 5/RConn1 -- Three-Phase Series RLC B2_G3/RConn1
  Three-Phase Fault10/LConn3 -- SM 12/LConn3 -- Three-Phase Series RLC B6_L14/LConn3
  Three-Phase Fault10/LConn2 -- SM 12/LConn2 -- Three-Phase Series RLC B6_L14/LConn2
  Three-Phase Fault10/LConn1 -- SM 12/LConn1 -- Three-Phase Series RLC B6_L14/LConn1
  Three-Phase Series RLC B6_L13_2/LConn3 -- SM 10/LConn3 -- Three-Phase Fault9/LConn3
  Three-Phase Series RLC B6_L13_2/LConn2 -- SM 10/LConn2 -- Three-Phase Fault9/LConn2
  Three-Phase Series RLC B6_L13_2/LConn1 -- SM 10/LConn1 -- Three-Phase Fault9/LConn1
  Three-Phase Series RLC B6_L13/RConn3 -- SM 8/LConn3 -- Three-Phase Fault7/LConn3
  Three-Phase Series RLC B6_L13/RConn2 -- SM 8/LConn2 -- Three-Phase Fault7/LConn2
  Three-Phase Fault7/LConn1 -- SM 8/LConn1 -- Three-Phase Series RLC B6_L13/RConn1
  Three-Phase Fault8/LConn3 -- SM 7/LConn3 -- Three-Phase Series RLC B6_L12/LConn3
  Three-Phase Fault8/LConn2 -- SM 7/LConn2 -- Three-Phase Series RLC B6_L12/LConn2
  Three-Phase Fault8/LConn1 -- SM 7/LConn1 -- Three-Phase Series RLC B6_L12/LConn1
  Three-Phase Fault11/LConn3 -- SM 11/LConn3 -- Three-Phase Series RLC B6_L10/LConn3
  Three-Phase Series RLC B6_L10/LConn2 -- SM 11/LConn2 -- Three-Phase Fault11/LConn2
  Three-Phase Series RLC B6_L10/LConn1 -- SM 11/LConn1 -- Three-Phase Fault11/LConn1
  Three-Phase Series RLC B8_L10/LConn3 -- SM 15/LConn3 -- Three-Phase Fault13/LConn3
  Three-Phase Fault13/LConn2 -- SM 15/LConn2 -- Three-Phase Series RLC B8_L10/LConn2
  Three-Phase Fault13/LConn1 -- SM 15/LConn1 -- Three-Phase Series RLC B8_L10/LConn1
  Three-Phase Fault12/LConn3 -- SM 14/LConn3 -- Three-Phase Series RLC B8_L14/LConn3
  Three-Phase Fault12/LConn2 -- SM 14/LConn2 -- Three-Phase Series RLC B8_L14/LConn2
  Three-Phase Series RLC B8_L14/LConn1 -- SM 14/LConn1 -- Three-Phase Fault12/LConn1
  Three-Phase V-I Measurement L9/LConn2 -- Three-Phase V-I Measurement3/RConn2 -- SM 15/RConn2 -- SM 14/RConn2 -- Three-Phase V-I Measurement1/RConn2
  Three-Phase V-I Measurement L9/LConn3 -- Three-Phase V-I Measurement3/RConn3 -- SM 15/RConn3 -- SM 14/RConn3 -- Three-Phase V-I Measurement1/RConn3
  Three-Phase V-I Measurement L11/LConn3 -- SM 11/RConn3 -- CB 7/LConn3
  Three-Phase V-I Measurement L11/LConn2 -- SM 11/RConn2 -- CB 7/LConn2
  Three-Phase V-I Measurement L11/LConn1 -- SM 11/RConn1 -- CB 7/LConn1
  Three-Phase V-I Measurement L11/RConn1 -- Three-Phase Series RLC Load11/LConn1 -- Load Flow Bus6/LConn1
  Three-Phase Series RLC Load11/LConn3 -- Three-Phase V-I Measurement L11/RConn3
  Three-Phase Series RLC Load11/LConn2 -- Three-Phase V-I Measurement L11/RConn2
  Three-Phase Transformer (Two Windings)3/RConn3 -- SM 13/LConn3 -- Three-Phase V-I Measurement2/RConn3
  Three-Phase Transformer (Two Windings)3/RConn2 -- Three-Phase V-I Measurement2/RConn2 -- SM 13/LConn2
  Three-Phase Fault6/LConn3 -- SM 9/LConn3 -- Three-Phase Series RLC B6_L11/LConn3
  Three-Phase Fault6/LConn2 -- SM 9/LConn2 -- Three-Phase Series RLC B6_L11/LConn2
  Three-Phase Fault6/LConn1 -- SM 9/LConn1 -- Three-Phase Series RLC B6_L11/LConn1
  SM 13/RConn2 -- Three-Phase Series RLC B8_L5/LConn2
  Load Flow Bus12/LConn1 -- Three-Phase V-I Measurement2/LConn1 -- Three-Phase Transformer (Two Windings)2/LConn1
  Three-Phase Series RLC Load9/LConn1 -- Three-Phase V-I Measurement L9/RConn1
  Three-Phase Series RLC Load9/LConn3 -- Three-Phase V-I Measurement L9/RConn3
  Three-Phase Series RLC Load9/LConn2 -- Three-Phase V-I Measurement L9/RConn2
  Three-Phase Series RLC Load4/LConn1 -- Three-Phase V-I Measurement L4/RConn1
  Three-Phase Series RLC Load4/LConn2 -- Three-Phase V-I Measurement L4/RConn2
  Three-Phase Series RLC Load4/LConn3 -- Three-Phase V-I Measurement L4/RConn3
  Three-Phase Series RLC B1_L4/LConn3 -- SM 1/LConn3 -- Three-Phase Fault5/LConn3
  Three-Phase Series RLC B1_L4/LConn2 -- SM 1/LConn2 -- Three-Phase Fault5/LConn2
  Three-Phase Series RLC B1_L4/LConn1 -- SM 1/LConn1 -- Three-Phase Fault5/LConn1
  Three-Phase V-I Measurement OutG6/RConn1 -- Three-Phase V-I Measurement/RConn1 -- SM 9/RConn1 -- SM 7/RConn1 -- SM 8/RConn1
  Three-Phase V-I Measurement OutG6/RConn2 -- Three-Phase V-I Measurement/RConn2 -- SM 9/RConn2 -- SM 7/RConn2 -- SM 8/RConn2
  SM 9/RConn3 -- SM 7/RConn3 -- SM 8/RConn3 -- Three-Phase V-I Measurement/RConn3 -- Three-Phase V-I Measurement OutG6/RConn3
  Three-Phase V-I Measurement G6/RConn3 -- Three-Phase V-I Measurement L6/LConn3 -- Three-Phase V-I Measurement OutG6/LConn3
  Three-Phase V-I Measurement G6/RConn1 -- Load Flow Bus5/LConn1 -- Three-Phase V-I Measurement OutG6/LConn1 -- Three-Phase V-I Measurement L6/LConn1
  Three-Phase V-I Measurement OutG6/LConn2 -- Three-Phase V-I Measurement G6/RConn2 -- Three-Phase V-I Measurement L6/LConn2
  Three-Phase Series RLC Load6/LConn3 -- Three-Phase V-I Measurement L6/RConn3
  Three-Phase Series RLC Load6/LConn1 -- Three-Phase V-I Measurement L6/RConn1
  Three-Phase Series RLC Load6/LConn2 -- Three-Phase V-I Measurement L6/RConn2
  Three-Phase V-I Measurement G6/LConn3 -- Three-Phase Breaker6/RConn3
  Three-Phase V-I Measurement G6/LConn2 -- Three-Phase Breaker6/RConn2
  Three-Phase V-I Measurement G6/LConn1 -- Three-Phase Breaker6/RConn1
  Three-Phase V-I Measurement L5/LConn1 -- Three-Phase Series RLC Load5/LConn1 -- Load Flow Bus2/LConn1
  Three-Phase Series RLC Load5/LConn3 -- Three-Phase V-I Measurement L5/LConn3
  Three-Phase Series RLC Load5/LConn2 -- Three-Phase V-I Measurement L5/LConn2
  Three-Phase V-I Measurement L5/RConn2 -- SM 1/RConn2 -- Three-Phase Transformer (Two Windings)/RConn2 -- CB 3/LConn2 -- CB 0/LConn2
  Three-Phase Fault4/LConn3 -- SM 0/LConn3 -- Three-Phase Series RLC B1_L5/LConn3
  Three-Phase Fault4/LConn2 -- SM 0/LConn2 -- Three-Phase Series RLC B1_L5/LConn2
  Three-Phase Series RLC B1_L5/LConn1 -- SM 0/LConn1 -- Three-Phase Fault4/LConn1
  SM 0/RConn3 -- Three-Phase V-I Measurement G1/RConn3 -- CB 2/LConn3
  Three-Phase V-I Measurement G1/RConn1 -- CB 2/LConn1 -- SM 0/RConn1
  Three-Phase V-I Measurement G1/RConn2 -- CB 2/LConn2 -- SM 0/RConn2
  Three-Phase Fault1/LConn3 -- SM 4/LConn3 -- Three-Phase Series RLC B2_L4/LConn3
  Three-Phase Fault1/LConn2 -- SM 4/LConn2 -- Three-Phase Series RLC B2_L4/LConn2
  Three-Phase Fault1/LConn1 -- SM 4/LConn1 -- Three-Phase Series RLC B2_L4/LConn1
  Three-Phase Series RLC Load3/LConn2 -- Three-Phase V-I Measurement L3/RConn2
  Three-Phase Series RLC Load3/LConn3 -- Three-Phase V-I Measurement L3/RConn3
  Three-Phase Series RLC Load3/LConn1 -- Three-Phase V-I Measurement L3/RConn1
  Three-Phase V-I Measurement OutG3/LConn1 -- Load Flow Bus3/LConn1 -- Three-Phase V-I Measurement G3/RConn1 -- Three-Phase V-I Measurement L3/LConn1
  Three-Phase V-I Measurement OutG3/LConn2 -- Three-Phase V-I Measurement L3/LConn2 -- Three-Phase V-I Measurement G3/RConn2
  Three-Phase V-I Measurement OutG3/LConn3 -- Three-Phase V-I Measurement L3/LConn3 -- Three-Phase V-I Measurement G3/RConn3
  Three-Phase V-I Measurement G3/LConn3 -- Three-Phase Breaker3/RConn3
  Three-Phase V-I Measurement G3/LConn2 -- Three-Phase Breaker3/RConn2
  Three-Phase V-I Measurement G3/LConn1 -- Three-Phase Breaker3/RConn1
  Three-Phase V-I Measurement OutG3/RConn3 -- SM 6/RConn3 -- CB 5/LConn3
  Three-Phase V-I Measurement OutG3/RConn2 -- SM 6/RConn2 -- CB 5/LConn2
  Three-Phase V-I Measurement OutG3/RConn1 -- SM 6/RConn1 -- CB 5/LConn1
  Three-Phase Fault15/LConn1 -- SM 6/LConn1 -- Three-Phase Series RLC B3_L4/LConn1
  Three-Phase Fault15/LConn3 -- SM 6/LConn3 -- Three-Phase Series RLC B3_L4/LConn3
  Three-Phase Fault15/LConn2 -- SM 6/LConn2 -- Three-Phase Series RLC B3_L4/LConn2
  Load Flow Bus1/LConn1 -- Three-Phase V-I Measurement OutG2/RConn1 -- SM 5/RConn1 -- SM 4/RConn1 -- SM 2/RConn1 -- SM 3/RConn1
  Three-Phase V-I Measurement OutG2/RConn2 -- SM 5/RConn2 -- SM 4/RConn2 -- SM 2/RConn2 -- SM 3/RConn2
  Three-Phase V-I Measurement OutG2/RConn3 -- SM 5/RConn3 -- SM 4/RConn3 -- SM 3/RConn3 -- SM 2/RConn3
  Three-Phase V-I Measurement G2/LConn3 -- Three-Phase Breaker1/RConn3
  Three-Phase V-I Measurement G2/LConn2 -- Three-Phase Breaker1/RConn2
  Three-Phase V-I Measurement G2/LConn1 -- Three-Phase Breaker1/RConn1
  Three-Phase Fault2/LConn3 -- SM 3/LConn3 -- Three-Phase Series RLC B2_L5/LConn3
  Three-Phase Fault2/LConn2 -- SM 3/LConn2 -- Three-Phase Series RLC B2_L5/LConn2
  Three-Phase Fault2/LConn1 -- SM 3/LConn1 -- Three-Phase Series RLC B2_L5/LConn1
  Three-Phase Fault/LConn3 -- SM 5/LConn3 -- Three-Phase Series RLC B2_G3/LConn3
  Three-Phase Fault/LConn2 -- SM 5/LConn2 -- Three-Phase Series RLC B2_G3/LConn2
  Three-Phase Fault/LConn1 -- SM 5/LConn1 -- Three-Phase Series RLC B2_G3/LConn1
  Three-Phase V-I Measurement L2/LConn3 -- Three-Phase V-I Measurement G2/RConn3 -- Three-Phase V-I Measurement OutG2/LConn3
  Three-Phase Fault3/LConn3 -- SM 2/LConn3 -- Three-Phase Series RLC B2_G1/LConn3
  Three-Phase Fault3/LConn2 -- SM 2/LConn2 -- Three-Phase Series RLC B2_G1/LConn2
  Three-Phase Fault3/LConn1 -- SM 2/LConn1 -- Three-Phase Series RLC B2_G1/LConn1
  Three-Phase Series RLC Load2/LConn1 -- Three-Phase V-I Measurement L2/RConn1
  Three-Phase Series RLC Load2/LConn3 -- Three-Phase V-I Measurement L2/RConn3
  Three-Phase Series RLC Load2/LConn2 -- Three-Phase V-I Measurement L2/RConn2
  Three-Phase Source2/RConn1 -- Load Flow Bus14/LConn1 -- Three-Phase Breaker1/LConn1
  Three-Phase Source2/RConn3 -- Three-Phase Breaker1/LConn3
  Three-Phase Source2/RConn2 -- Three-Phase Breaker1/LConn2
  Three-Phase Series RLC Load14/LConn1 -- Three-Phase V-I Measurement L14/RConn1
  Three-Phase Series RLC Load14/LConn2 -- Three-Phase V-I Measurement L14/RConn2
  Three-Phase Series RLC Load14/LConn3 -- Three-Phase V-I Measurement L14/RConn3
  Three-Phase Series RLC Load13/LConn2 -- Three-Phase V-I Measurement L13/RConn2
  Three-Phase Series RLC Load13/LConn1 -- Three-Phase V-I Measurement L13/RConn1
  Three-Phase Series RLC Load13/LConn3 -- Three-Phase V-I Measurement L13/RConn3
  Three-Phase Series RLC Load12/LConn1 -- Three-Phase V-I Measurement L12/RConn1
  Three-Phase Series RLC Load12/LConn2 -- Three-Phase V-I Measurement L12/RConn2
  Three-Phase Series RLC Load12/LConn3 -- Three-Phase V-I Measurement L12/RConn3
  Three-Phase Series RLC Load10/LConn1 -- Three-Phase V-I Measurement L10/RConn1
  Three-Phase Series RLC Load10/LConn2 -- Three-Phase V-I Measurement L10/RConn2
  Three-Phase Series RLC Load10/LConn3 -- Three-Phase V-I Measurement L10/RConn3
  Three-Phase Source6/RConn3 -- Three-Phase Breaker6/LConn3
  Three-Phase Source6/RConn2 -- Three-Phase Breaker6/LConn2
  Three-Phase Source6/RConn1 -- Load Flow Bus15/LConn1 -- Three-Phase Breaker6/LConn1
  Three-Phase Source3/RConn3 -- Three-Phase Breaker3/LConn3
  Three-Phase Source3/RConn2 -- Three-Phase Breaker3/LConn2
  Three-Phase Source3/RConn1 -- Load Flow Bus18/LConn1 -- Three-Phase Breaker3/LConn1
  Three-Phase V-I Measurement L12/LConn1 -- SM 10/RConn1 -- CB 8/LConn1 -- Load Flow Bus7/LConn1
  SM 10/RConn2 -- Three-Phase V-I Measurement L12/LConn2 -- CB 8/LConn2
  Three-Phase Transformer (Two Windings)1/RConn3 -- CB 6/LConn3 -- CB 1/LConn3 -- CB 4/LConn3 -- Three-Phase V-I Measurement L4/LConn3 -- Three-Phase Transformer (Two Windings)2/RConn3
  CB 9/LConn3 -- CB 10/LConn3 -- SM 12/RConn3 -- Three-Phase V-I Measurement L13/LConn3
  CB 9/LConn2 -- CB 10/LConn2 -- SM 12/RConn2 -- Three-Phase V-I Measurement L13/LConn2
  Load Flow Bus4/LConn1 -- CB 6/LConn1 -- CB 4/LConn1 -- CB 1/LConn1 -- Three-Phase Transformer (Two Windings)1/RConn1 -- Three-Phase V-I Measurement L4/LConn1 -- Three-Phase Transformer (Two Windings)2/RConn1
  CB 8/LConn3 -- SM 10/RConn3 -- Three-Phase V-I Measurement L12/LConn3
  Three-Phase Transformer (Two Windings)1/RConn2 -- CB 6/LConn2 -- CB 4/LConn2 -- CB 1/LConn2 -- Three-Phase V-I Measurement L4/LConn2 -- Three-Phase Transformer (Two Windings)2/RConn2
  Load Flow Bus8/LConn1 -- SM 12/RConn1 -- CB 9/LConn1 -- CB 10/LConn1 -- Three-Phase V-I Measurement L13/LConn1
  Three-Phase V-I Measurement L5/RConn3 -- SM 1/RConn3 -- CB 3/LConn3 -- CB 0/LConn3 -- Three-Phase Transformer (Two Windings)/RConn3
  Three-Phase Transformer (Two Windings)/RConn1 -- SM 1/RConn1 -- CB 0/LConn1 -- CB 3/LConn1 -- Three-Phase V-I Measurement L5/RConn1
  Three-Phase V-I Measurement L2/LConn1 -- Three-Phase V-I Measurement OutG2/LConn1 -- Three-Phase V-I Measurement G2/RConn1
  Three-Phase V-I Measurement G2/RConn2 -- Three-Phase V-I Measurement OutG2/LConn2 -- Three-Phase V-I Measurement L2/LConn2
  Three-Phase Source8/RConn2 -- Three-Phase Breaker/LConn2
  Three-Phase Breaker/RConn1 -- Three-Phase V-I Measurement G8/RConn1
  Three-Phase Breaker/RConn2 -- Three-Phase V-I Measurement G8/RConn2
  Three-Phase Source8/RConn1 -- Load Flow Bus16/LConn1 -- Three-Phase Breaker/LConn1
  Three-Phase Breaker/RConn3 -- Three-Phase V-I Measurement G8/RConn3
  Three-Phase Source8/RConn3 -- Three-Phase Breaker/LConn3
  Load Flow Bus10/LConn1 -- CB 15/LConn1 -- CB 11/LConn1 -- Three-Phase V-I Measurement L10/LConn1
  Three-Phase V-I Measurement L9/LConn1 -- Three-Phase V-I Measurement1/RConn1 -- Three-Phase V-I Measurement3/RConn1 -- SM 15/RConn1 -- SM 14/RConn1
  Load Flow Bus13/LConn1 -- CB 13/LConn1 -- Three-Phase V-I Measurement G8/LConn1
  Load Flow Bus9/LConn1 -- CB 14/LConn1 -- CB 12/LConn1 -- Three-Phase V-I Measurement L14/LConn1
  SM 13/RConn1 -- Three-Phase Series RLC B8_L5/LConn1
  SM 13/RConn3 -- Three-Phase Series RLC B8_L5/LConn3
